simulink library "ESTS_FRIC_HILO_PREPROC"  (R2024b)
settings: Solver=VariableStepAuto  StartTime=0.0  StopTime=10.0  RelTol=1e-3
undefined symbols (not defined in the file or in its folder): ESTS_FRIC_HILO_PREPROC_p_ALatHiLim_mps2, ESTS_FRIC_HILO_PREPROC_p_ALatLoLim_mps2, ESTS_FRIC_HILO_PREPROC_p_ALgtHiLim_mps2, ESTS_FRIC_HILO_PREPROC_p_ALgtLoLim_mps2, ESTS_FRIC_HILO_PREPROC_p_SlipHiLim_p1, ESTS_FRIC_HILO_PREPROC_p_SlipLoLim_p1, ESTS_FRIC_HILO_PREPROC_p_SpdLim_mps, ESTS_FRIC_HILO_PREPROC_p_TqHiLim_Nm, ESTS_FRIC_HILO_PREPROC_p_TqLoLim_Nm
settings Model: Creator=blatak  LastModifiedBy=blatak

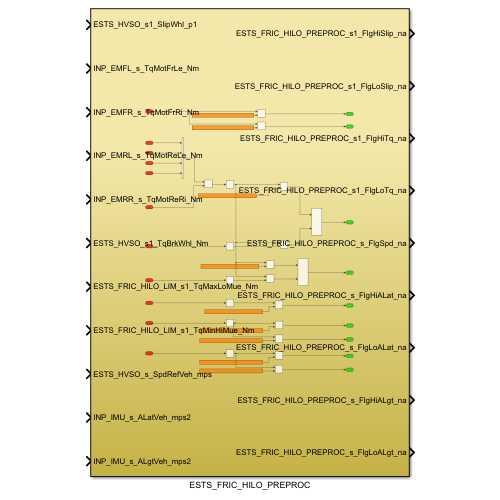
[thumbnail: Simulink's stored preview of the top-level diagram]
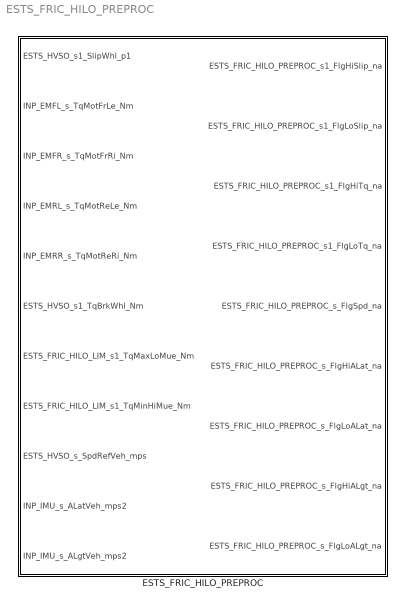
== system ESTS_FRIC_HILO_PREPROC ==
  ESTS_FRIC_HILO_PREPROC : Subsystem

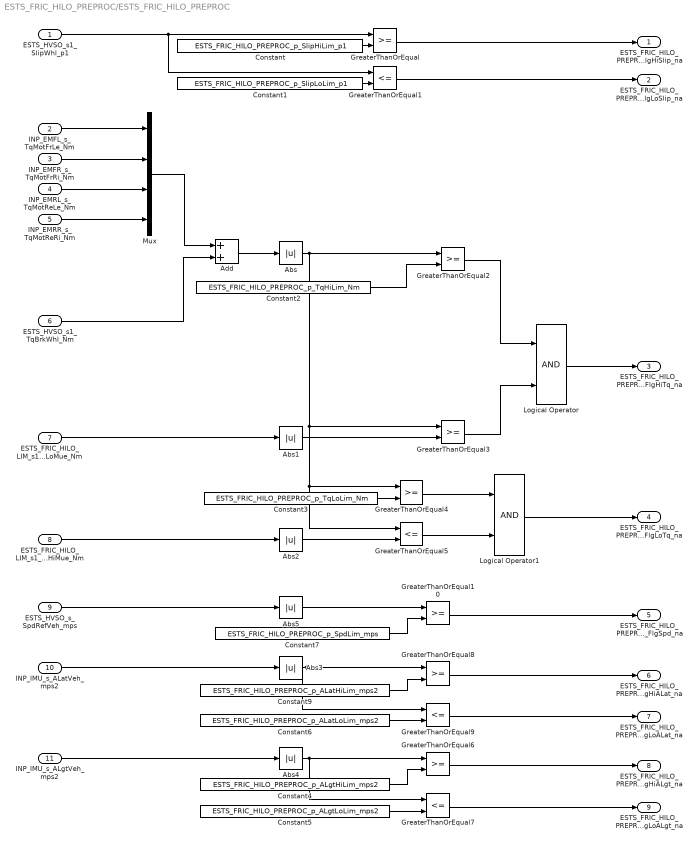
== system ESTS_FRIC_HILO_PREPROC/ESTS_FRIC_HILO_PREPROC ==
  ESTS_HVSO_s1_SlipWhl_p1 : Inport
  INP_EMFL_s_TqMotFrLe_Nm : Inport  Port=2
  INP_EMFR_s_TqMotFrRi_Nm : Inport  Port=3
  INP_EMRL_s_TqMotReLe_Nm : Inport  Port=4
  INP_EMRR_s_TqMotReRi_Nm : Inport  Port=5
  ESTS_HVSO_s1_TqBrkWhl_Nm : Inport  Port=6
  ESTS_FRIC_HILO_LIM_s1_TqMaxLoMue_Nm : Inport  Port=7
  ESTS_FRIC_HILO_LIM_s1_TqMinHiMue_Nm : Inport  Port=8
  ESTS_HVSO_s_SpdRefVeh_mps : Inport  Port=9
  INP_IMU_s_ALatVeh_mps2 : Inport  Port=10
  INP_IMU_s_ALgtVeh_mps2 : Inport  Port=11
  Abs{,1..5} (6 alike) : Abs  SaturateOnIntegerOverflow=off
  Add : Sum
  Constant : Constant  Value=ESTS_FRIC_HILO_PREPROC_p_SlipHiLim_p1
  Constant1 : Constant  Value=ESTS_FRIC_HILO_PREPROC_p_SlipLoLim_p1
  Constant2 : Constant  Value=ESTS_FRIC_HILO_PREPROC_p_TqHiLim_Nm
  Constant3 : Constant  Value=ESTS_FRIC_HILO_PREPROC_p_TqLoLim_Nm
  Constant4 : Constant  Value=ESTS_FRIC_HILO_PREPROC_p_ALgtHiLim_mps2
  Constant5 : Constant  Value=ESTS_FRIC_HILO_PREPROC_p_ALgtLoLim_mps2
  Constant6 : Constant  Value=ESTS_FRIC_HILO_PREPROC_p_ALatLoLim_mps2
  Constant7 : Constant  Value=ESTS_FRIC_HILO_PREPROC_p_SpdLim_mps
  Constant9 : Constant  Value=ESTS_FRIC_HILO_PREPROC_p_ALatHiLim_mps2
  GreaterThanOrEqual{,2..4,6,8,10} (7 alike) : RelationalOperator  OutDataTypeStr=boolean  RndMeth=Simplest  InputSameDT=off
  GreaterThanOrEqual{1,5,7,9} (4 alike) : RelationalOperator  Operator=<=  OutDataTypeStr=boolean  RndMeth=Simplest  InputSameDT=off
  Logical Operator : Logic  AllPortsSameDT=off  OutDataTypeStr=boolean
  Logical Operator1 : Logic  AllPortsSameDT=off  OutDataTypeStr=boolean
  Mux : Mux
  ESTS_FRIC_HILO_PREPROC_s1_FlgHiSlip_na : Outport
  ESTS_FRIC_HILO_PREPROC_s1_FlgLoSlip_na : Outport  Port=2
  ESTS_FRIC_HILO_PREPROC_s1_FlgHiTq_na : Outport  Port=3
  ESTS_FRIC_HILO_PREPROC_s1_FlgLoTq_na : Outport  Port=4
  ESTS_FRIC_HILO_PREPROC_s_FlgSpd_na : Outport  Port=5
  ESTS_FRIC_HILO_PREPROC_s_FlgHiALat_na : Outport  Port=6
  ESTS_FRIC_HILO_PREPROC_s_FlgLoALat_na : Outport  Port=7
  ESTS_FRIC_HILO_PREPROC_s_FlgHiALgt_na : Outport  Port=8
  ESTS_FRIC_HILO_PREPROC_s_FlgLoALgt_na : Outport  Port=9
  wires:
  GreaterThanOrEqual6/1 -> ESTS_FRIC_HILO_PREPROC_s_FlgHiALgt_na/1
  ESTS_HVSO_s_SpdRefVeh_mps/1 -> Abs5/1
  GreaterThanOrEqual7/1 -> ESTS_FRIC_HILO_PREPROC_s_FlgLoALgt_na/1
  Constant1/1 -> GreaterThanOrEqual1/2
  Logical Operator1/1 -> ESTS_FRIC_HILO_PREPROC_s1_FlgLoTq_na/1
  INP_IMU_s_ALatVeh_mps2/1 -> Abs3/1
  Abs/1 -> GreaterThanOrEqual5/1, GreaterThanOrEqual4/1, GreaterThanOrEqual3/1, GreaterThanOrEqual2/1
  INP_IMU_s_ALgtVeh_mps2/1 -> Abs4/1
  Logical Operator/1 -> ESTS_FRIC_HILO_PREPROC_s1_FlgHiTq_na/1
  ESTS_HVSO_s1_SlipWhl_p1/1 -> GreaterThanOrEqual/1, GreaterThanOrEqual1/1
  GreaterThanOrEqual/1 -> ESTS_FRIC_HILO_PREPROC_s1_FlgHiSlip_na/1
  GreaterThanOrEqual4/1 -> Logical Operator1/1
  ESTS_FRIC_HILO_LIM_s1_TqMinHiMue_Nm/1 -> Abs2/1
  ESTS_HVSO_s1_TqBrkWhl_Nm/1 -> Add/2
  GreaterThanOrEqual10/1 -> ESTS_FRIC_HILO_PREPROC_s_FlgSpd_na/1
  Constant2/1 -> GreaterThanOrEqual2/2
  Add/1 -> Abs/1
  GreaterThanOrEqual5/1 -> Logical Operator1/2
  INP_EMRL_s_TqMotReLe_Nm/1 -> Mux/3
  ESTS_FRIC_HILO_LIM_s1_TqMaxLoMue_Nm/1 -> Abs1/1
  Constant/1 -> GreaterThanOrEqual/2
  Constant5/1 -> GreaterThanOrEqual7/2
  Abs1/1 -> GreaterThanOrEqual3/2
  Abs4/1 -> GreaterThanOrEqual7/1, GreaterThanOrEqual6/1
  Mux/1 -> Add/1
  INP_EMRR_s_TqMotReRi_Nm/1 -> Mux/4
  GreaterThanOrEqual1/1 -> ESTS_FRIC_HILO_PREPROC_s1_FlgLoSlip_na/1
  INP_EMFL_s_TqMotFrLe_Nm/1 -> Mux/1
  INP_EMFR_s_TqMotFrRi_Nm/1 -> Mux/2
  Constant7/1 -> GreaterThanOrEqual10/2
  Constant4/1 -> GreaterThanOrEqual6/2
  GreaterThanOrEqual3/1 -> Logical Operator/2
  GreaterThanOrEqual2/1 -> Logical Operator/1
  Constant3/1 -> GreaterThanOrEqual4/2
  Abs2/1 -> GreaterThanOrEqual5/2
  Constant9/1 -> GreaterThanOrEqual8/2
  Constant6/1 -> GreaterThanOrEqual9/2
  GreaterThanOrEqual9/1 -> ESTS_FRIC_HILO_PREPROC_s_FlgLoALat_na/1
  GreaterThanOrEqual8/1 -> ESTS_FRIC_HILO_PREPROC_s_FlgHiALat_na/1
  Abs3/1 -> GreaterThanOrEqual8/1, GreaterThanOrEqual9/1
  Abs5/1 -> GreaterThanOrEqual10/1
